simulink model "PID_SimulationModel"  (R2023b)
settings: Solver=VariableStepAuto  StartTime=0.0  StopTime=20  RelTol=1e-3
settings Model: Creator=joser  LastModifiedBy=joser

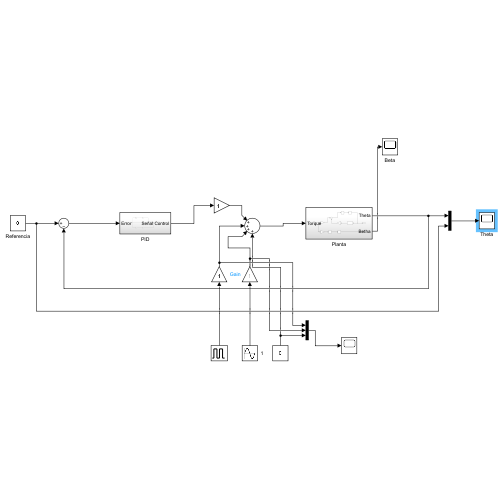
[thumbnail: Simulink's stored preview of the top-level diagram]
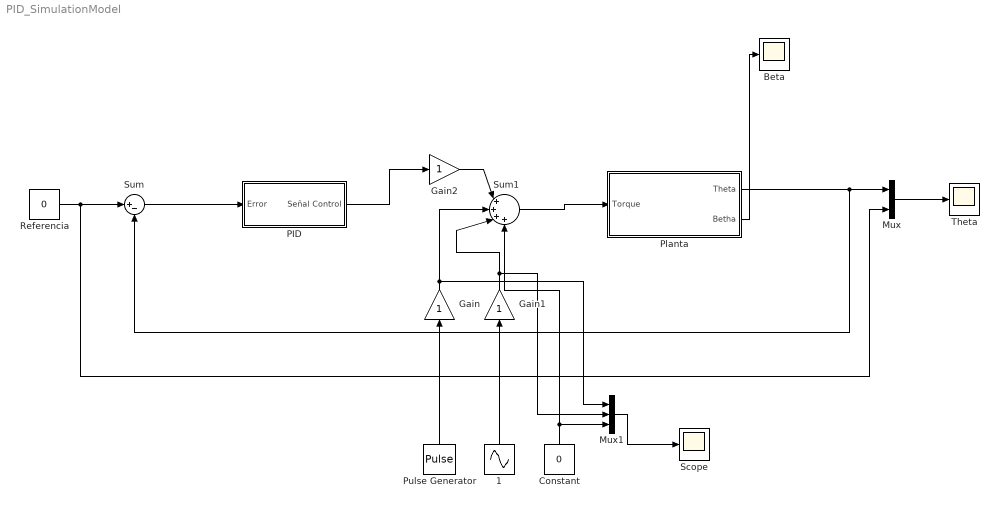
== system PID_SimulationModel ==
  1 : Sin  Amplitude=10  Frequency=50  SampleTime=0
  Beta : Scope
  Constant : Constant  Value=0
  Gain : Gain
  Gain1 : Gain
  Gain2 : Gain
  Mux : Mux  Inputs=2
  Mux1 : Mux  Inputs=3
  PID : Subsystem
  Planta : Subsystem
  Pulse Generator : DiscretePulseGenerator  PulseType=Time based  Amplitude=20  Period=3  PulseWidth=5
  Referencia : Constant  Value=0
  Scope : Scope
  Sum : Sum  Inputs=|+-
  Sum1 : Sum  Inputs=|++++
  Theta : Scope
  wires:
  Planta/1(Theta) -> Sum/2, Mux/1
  Referencia/1 -> Mux/2, Sum/1
  Planta/2(Betha) -> Beta/1
  Mux/1 -> Theta/1
  Sum1/1 -> Planta/1(Torque)
  Sum/1 -> PID/1(Error)
  Pulse Generator/1 -> Gain/1
  Gain/1 -> Sum1/2, Mux1/1
  1/1 -> Gain1/1
  Gain1/1 -> Sum1/3, Mux1/2
  Mux1/1 -> Scope/1
  PID/1(Señal Control) -> Gain2/1
  Constant/1 -> Sum1/4, Mux1/3
  Gain2/1 -> Sum1/1

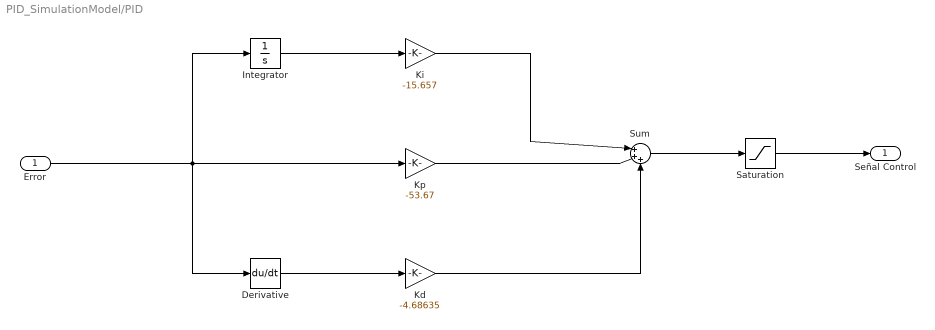
== system PID_SimulationModel/PID ==
  Error : Inport
  Derivative : Derivative
  Integrator : Integrator
  Kd : Gain  Gain=-4.68635
  Ki : Gain  Gain=-15.657
  Kp : Gain  Gain=-53.67
  Saturation : Saturate  UpperLimit=100  LowerLimit=-100
  Sum : Sum  Inputs=|+++
  Señal Control : Outport
  wires:
  Ki/1 -> Sum/1
  Kp/1 -> Sum/2
  Kd/1 -> Sum/3
  Integrator/1 -> Ki/1
  Error/1 -> Derivative/1, Integrator/1, Kp/1
  Derivative/1 -> Kd/1
  Sum/1 -> Saturation/1
  Saturation/1 -> Señal Control/1

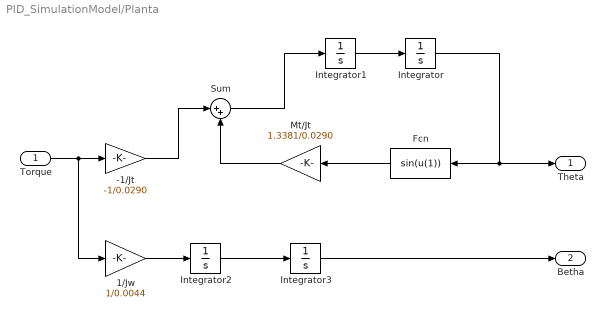
== system PID_SimulationModel/Planta ==
  Torque : Inport
  -1/Jt : Gain  Gain=-1/0.0290
  1/Jw : Gain  Gain=1/0.0044
  Fcn : Fcn  Expr=sin(u(1))
  Integrator : Integrator  InitialCondition=pi  WrapState=on
  Integrator1 : Integrator
  Integrator2 : Integrator
  Integrator3 : Integrator  WrapState=on  WrappedStateUpperValue=2*pi  WrappedStateLowerValue=0
  Mt/Jt : Gain  Gain=1.3381/0.0290
  Sum : Sum  Inputs=|++
  Theta : Outport
  Betha : Outport  Port=2
  wires:
  Torque/1 -> 1/Jw/1, -1/Jt/1
  -1/Jt/1 -> Sum/1
  Mt/Jt/1 -> Sum/2
  Integrator/1 -> Theta/1, Fcn/1
  Integrator1/1 -> Integrator/1
  Sum/1 -> Integrator1/1
  Fcn/1 -> Mt/Jt/1
  Integrator2/1 -> Integrator3/1
  Integrator3/1 -> Betha/1
  1/Jw/1 -> Integrator2/1
